simulink model "two_legged_raibert_hopper"  (R2014a)
settings: Solver=FixedStepDiscrete  StartTime=0.0  StopTime=inf  FixedStep=sample_time  RelTol=1e-3
undefined symbols (not defined in the file): A1_notch_f1, A2_notch_f1, A_lpf_accel, A_lpf_dtau, B1_lpf_accel, B1_lpf_dtau, B1_notch_f1, B2_lpf_accel, B2_lpf_dtau, B2_notch_f1, boom_height, boom_mount_angle, boom_mount_to_center_diagonal, boom_mount_to_com, contact_threshold, control_start_time, desired_torso_angle, DiscIntNeverNeededParam, dt_thrust, dx_avg_desired, dx_avg_samples, dx_desired_step, extra_leg_damping, F_thrust, fcut_contact, g, i_limit_lateral, initial_dt, j_segments, k_ff, K_notch_f1, k_placement, k_sea, kd_flight, kd_lateral, kd_leg_angle, kd_leg_length_secondary, kd_sea_torque_flight, kd_sea_torque_stance, kd_torso, kd_virtual, ki_lateral, kp_flight_max, kp_flight_min, kp_lateral, kp_leg_angle, kp_leg_length_secondary, kp_sea_torque_flight, kp_sea_torque_stance, kp_torso, kp_virtual, l0_virtual, l_boom, l_max, l_min, l_retract, l_seg, lambda1, lambda2, lateral_offset ... (+20)
libraries: simulink x14
(part 1 of 2)
settings Model: xpc_rtwmakecfg_data=_xpcethercatlib_  BufferReuse=off  Creator=wmartin  LastModifiedBy=wmartin
settings SolverCC: EnableConcurrentExecution=on
settings DataIOCC: MaxDataPoints=1000000000  SaveFormat=StructureWithTime
settings OptimizationCC: BlockReduction=off  OptimizeBlockIOStorage=off  BufferReuse=off  GlobalBufferReuse=off  ExpressionFolding=off  ExpressionDepthLimit=2147483647  LocalBlockOutputs=off
settings DebuggingCC: UnderspecifiedInitializationDetection=Classic  StateNameClashWarn=warning
settings HardwareCC: ProdIntDivRoundTo=Zero  ProdEndianess=LittleEndian  ProdHWDeviceType=Generic->32-bit x86 compatible
settings RTWCC: SystemTargetFile=slrt.tlc  TemplateMakefile=slrt_default_tmf  Description=Simulink Real-Time  RTWVerbose=off  ProcessScript=slrt_make_rtw_hook  RTWCompilerOptimization=On
settings SimulinkRealTimeCC: GeneratePreprocessorConditionals=Disable all  EnableShiftOperators=on  RL32LogBufSizeModifier=100000000

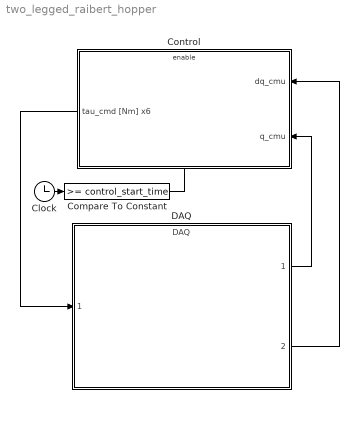
== system two_legged_raibert_hopper ==
  Clock : Clock
  Compare To Constant : simulink/Logic and Bit Operations/Compare To Constant  relop=>=  const=control_start_time  OutDataTypeStr=boolean
  Control : Subsystem
  DAQ : ModelReference  ModelNameDialog=DAQ  SimulationMode=Normal  ModelReferenceVersion=1.1402  CopyOfModelName=DAQ  DefaultDataLogging=on
  wires:
  DAQ/1 -> Control/2(q_cmu)
  DAQ/2 -> Control/1(dq_cmu)
  Clock/1 -> Compare To Constant/1
  Compare To Constant/1 -> Control/Enable
  Control/1(tau_cmd [Nm] x6) -> DAQ/1

== system two_legged_raibert_hopper/Control ==
  dq_cmu : Inport
  q_cmu : Inport  Port=2
  Enable : EnablePort  StatesWhenEnabling=reset
  Actuator Control : Subsystem
  Behavior Control : Subsystem
  tau_cmd [Nm] x6 : Outport  InitialOutput=[0 0 0 0 0 0]
  wires:
  Behavior Control/1(motor_torque_cmd) -> Actuator Control/1(tau_desired [Nm] x6)
  dq_cmu/1 -> Actuator Control/3(dq_cmu), Behavior Control/1(dq_cmu)
  Actuator Control/1(tau_cmd [Nm] x6) -> tau_cmd [Nm] x6/1
  q_cmu/1 -> Behavior Control/2(q_cmu), Actuator Control/2(q_cmu)

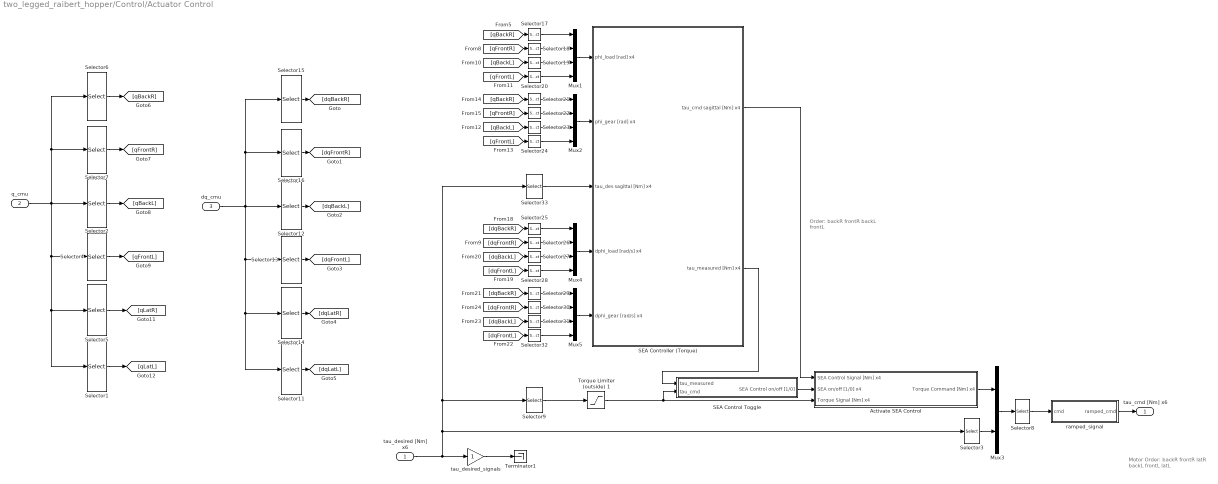
== system two_legged_raibert_hopper/Control/Actuator Control ==
  note: Motor Order:
      |
      | backR
      | frontR
      | latR
      | backL
      | frontL
      | latL
  note: Order:
      | backR
      | frontR
      | backL
      | frontL
  tau_desired [Nm] x6 : Inport
  q_cmu : Inport  Port=2
  dq_cmu : Inport  Port=3
  Activate SEA Control : Subsystem
  Mux{1..2,4..5} (4 alike) : Mux
  Mux3 : Mux  Inputs=2
  SEA Control Toggle : Subsystem
  SEA Controller (Torque) : Subsystem
  Selector1 : Selector  InputPortWidth=13  Indices=[10]
  Selector11 : Selector  InputPortWidth=13  Indices=[10]
  Selector12 : Selector  InputPortWidth=13  Indices=[5 6]
  Selector13 : Selector  InputPortWidth=13  Indices=[7 8]
  Selector14 : Selector  InputPortWidth=13  Indices=[9]
  Selector15 : Selector  InputPortWidth=13  Indices=[1 2]
  Selector16 : Selector  InputPortWidth=13  Indices=[3 4]
  Selector{17..20,25..28} (8 alike) : Selector  InputPortWidth=2  Indices=[1]
  Selector2 : Selector  InputPortWidth=13  Indices=[5 6]
  Selector{21..24,29..32} (8 alike) : Selector  InputPortWidth=2  Indices=[2]
  Selector3 : Selector  InputPortWidth=6  Indices=[3 6]
  Selector33 : Selector  InputPortWidth=6  Indices=[1 2 4 5]
  Selector4 : Selector  InputPortWidth=13  Indices=[7 8]
  Selector5 : Selector  InputPortWidth=13  Indices=[9]
  Selector6 : Selector  InputPortWidth=13  Indices=[1 2]
  Selector7 : Selector  InputPortWidth=13  Indices=[3 4]
  Selector8 : Selector  InputPortWidth=6  Indices=[1 2 5 3 4 6]
  Selector9 : Selector  InputPortWidth=6  Indices=[1 2 4 5]
  Terminator1 : Terminator
  Torque Limiter (outside) 1 : Saturate  UpperLimit=max_sagittal_unloaded_torque  LowerLimit=-max_sagittal_unloaded_torque
      settings: AttributesFormatString=Hi: %<UpperLimit>\nLo: %<LowerLimit>
  ramped_signal : Subsystem
  tau_desired_signals : Gain  Description=xPCTag(1)=tau_cmd_signal;
  tau_cmd [Nm] x6 : Outport  InitialOutput=[0 0 0 0 0 0]
  wires:
  Mux3/1 -> Selector8/1
  Selector3/1 -> Mux3/2
  Selector33/1 -> SEA Controller (Torque)/3(tau_des sagittal [Nm] x4)
  [dqFrontL] -> Selector32/1
  [dqBackL] -> Selector31/1
  [dqFrontR] -> Selector30/1
  Selector32/1 -> Mux5/4
  Selector30/1 -> Mux5/2
  Selector31/1 -> Mux5/3
  Selector29/1 -> Mux5/1
  [dqBackR] -> Selector29/1
  Mux5/1 -> SEA Controller (Torque)/5(dphi_gear [rad/s] x4)
  [dqFrontL] -> Selector28/1
  [dqBackL] -> Selector27/1
  [dqFrontR] -> Selector26/1
  Selector28/1 -> Mux4/4
  Selector26/1 -> Mux4/2
  Selector27/1 -> Mux4/3
  Selector25/1 -> Mux4/1
  [dqBackR] -> Selector25/1
  Mux4/1 -> SEA Controller (Torque)/4(dphi_load [rad/s] x4)
  [qFrontL] -> Selector24/1
  [qBackL] -> Selector23/1
  [qFrontR] -> Selector22/1
  Selector24/1 -> Mux2/4
  Selector22/1 -> Mux2/2
  Selector23/1 -> Mux2/3
  Selector21/1 -> Mux2/1
  [qBackR] -> Selector21/1
  Mux2/1 -> SEA Controller (Torque)/2(phi_gear [rad] x4)
  [qFrontL] -> Selector20/1
  [qBackL] -> Selector19/1
  [qFrontR] -> Selector18/1
  Selector20/1 -> Mux1/4
  Selector18/1 -> Mux1/2
  Selector19/1 -> Mux1/3
  Selector17/1 -> Mux1/1
  [qBackR] -> Selector17/1
  Mux1/1 -> SEA Controller (Torque)/1(phi_load [rad] x4)
  Selector13/1 -> [dqFrontL]
  Selector12/1 -> [dqBackL]
  Selector16/1 -> [dqFrontR]
  Selector15/1 -> [dqBackR]
  Selector11/1 -> [dqLatL]
  Selector14/1 -> [dqLatR]
  dq_cmu/1 -> Selector11/1, Selector14/1, Selector13/1, Selector15/1, Selector16/1, Selector12/1
  Selector8/1 -> ramped_signal/1(cmd)
  q_cmu/1 -> Selector2/1, Selector7/1, Selector6/1, Selector4/1, Selector5/1, Selector1/1
  Selector4/1 -> [qFrontL]
  Selector2/1 -> [qBackL]
  Selector7/1 -> [qFrontR]
  Selector6/1 -> [qBackR]
  Selector1/1 -> [qLatL]
  Selector5/1 -> [qLatR]
  tau_desired_signals/1 -> Terminator1/1
  ramped_signal/1(ramped_cmd) -> tau_cmd [Nm] x6/1
  tau_desired [Nm] x6/1 -> Selector33/1, Selector9/1, Selector3/1, tau_desired_signals/1
  Activate SEA Control/1(Torque Command [Nm] x4) -> Mux3/1
  Torque Limiter (outside) 1/1 -> Activate SEA Control/3(Torque Signal [Nm] x4), SEA Control Toggle/2(tau_cmd)
  SEA Controller (Torque)/1(tau_cmd sagittal [Nm] x4) -> Activate SEA Control/1(SEA Control Signal [Nm] x4)
  SEA Control Toggle/1(SEA Control on/off [1/0]) -> Activate SEA Control/2("SEA on/off [1/0] x4 ")
  SEA Controller (Torque)/2(tau_measured [Nm] x4) -> SEA Control Toggle/1(tau_measured)
  Selector9/1 -> Torque Limiter (outside) 1/1

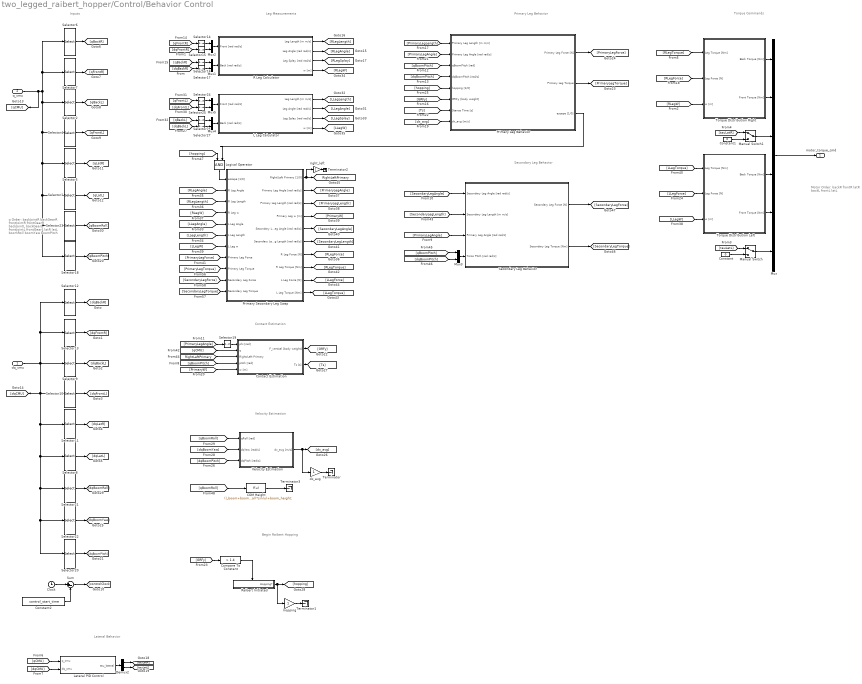
== system two_legged_raibert_hopper/Control/Behavior Control ==
  note: Motor Order:
      |
      | backR
      | frontR
      | latR
      | backL
      | frontL
      | latL
  note: q Order:
      |
      | backJointR
      | backGearR
      | frontJointR
      | frontGearR
      |
      | backJointL
      | backGearL
      | frontJointL
      | frontGearL
      |
      | latR
      | latL
      |
      | boomRoll
      | boomYaw
      | boomPitch
  note: Inputs
  note: Primary Leg Behavior
  note: Secondary Leg Behavior
  note: Torque Commands
  note: Lateral Behavior
  note: Leg Measurements
  note: Contact Estimation
  note: Velocity Estimation
  note: Begin Raibert Hopping
  dq_cmu : Inport
  q_cmu : Inport  Port=2
  COM Height : Fcn  Expr=(l_boom+boom_mount_to_center_diagonal)*sin(u)+boom_height;
  Clock : Clock
  Compare To Constant : simulink/Logic and Bit Operations/Compare To Constant  relop=>  const=1.4  OutDataTypeStr=boolean
  Constant : Constant  Value=0
  Constant1 : Constant  Value=0
  Constant2 : Constant  Value=control_start_time
  Contact Estimation : Subsystem
  Demux2 : Demux  Outputs=2
  L Leg Calculator : Subsystem
  Lateral PID Control : Subsystem
  Logical Operator : Logic  IconShape=distinctive  AllPortsSameDT=off  OutDataTypeStr=boolean
  Manual Switch : ManualSwitch
  Manual Switch1 : ManualSwitch
  Mux : Mux  Inputs=6
  Mux{1..5} (5 alike) : Mux  Inputs=2
  Primary Leg Behavior : Subsystem
  Primary Secondary Leg Swap : Subsystem
  R Leg Calculator : Subsystem
  Raibert Initiated : Subsystem
  Secondary Leg Behavior : Subsystem
  Selector1 : Selector  InputPortWidth=13  Indices=[10]
  Selector10 : Selector  InputPortWidth=13  Indices=[7 8]
  Selector11 : Selector  InputPortWidth=13  Indices=[9]
  Selector12 : Selector  InputPortWidth=13  Indices=[1 2]
  Selector13 : Selector  InputPortWidth=13  Indices=[3 4]
  Selector{14..17,19,24..27} (9 alike) : Selector  InputPortWidth=2  Indices=[1]
  Selector18 : Selector  InputPortWidth=13  Indices=[13]
  Selector2 : Selector  InputPortWidth=13  Indices=[5 6]
  Selector20 : Selector  InputPortWidth=13  Indices=[13]
  Selector21 : Selector  InputPortWidth=13  Indices=[11]
  Selector22 : Selector  InputPortWidth=13  Indices=[12]
  Selector23 : Selector  InputPortWidth=13  Indices=[11]
  Selector4 : Selector  InputPortWidth=13  Indices=[7 8]
  Selector5 : Selector  InputPortWidth=13  Indices=[9]
  Selector6 : Selector  InputPortWidth=13  Indices=[1 2]
  Selector7 : Selector  InputPortWidth=13  Indices=[3 4]
  Selector8 : Selector  InputPortWidth=13  Indices=[10]
  Selector9 : Selector  InputPortWidth=13  Indices=[5 6]
  Sum : Sum  Inputs=|+-
  Terminator{,1..3} (4 alike) : Terminator
  Torque Distribution Left : Subsystem
  Torque Distribution Right : Subsystem
  Velocity Estimation : Subsystem
  dx_avg : Gain
  hopping : Gain
  right_left : Gain
  motor_torque_cmd : Outport  OutputWhenDisabled=reset  InitialOutput=[0 0 0 0 0 0]
  tag scope: RightLeftPrimary=global
  wires:
  Lateral PID Control/1(tau_lateral) -> Demux2/1
  [dqCMU] -> Lateral PID Control/2(dq_cmu)
  [qCMU] -> Lateral PID Control/1(q_cmu)
  Sum/1 -> [controlClock]
  Selector4/1 -> [qFrontL]
  Selector2/1 -> [qBackL]
  Selector7/1 -> [qFrontR]
  Selector6/1 -> [qBackR]
  Selector1/1 -> [qLatL]
  Selector5/1 -> [qLatR]
  Constant2/1 -> Sum/2
  Clock/1 -> Sum/1
  Constant1/1 -> Manual Switch1/2
  Constant/1 -> Manual Switch/2
  Manual Switch/1 -> Mux/6
  Manual Switch1/1 -> Mux/3
  Mux/1 -> motor_torque_cmd/1
  Selector8/1 -> [dqLatL]
  Selector11/1 -> [dqLatR]
  Selector12/1 -> [dqBackR]
  Selector13/1 -> [dqFrontR]
  Selector9/1 -> [dqBackL]
  Selector10/1 -> [dqFrontL]
  [qBackR] -> Selector16/1
  [dqBackR] -> Selector17/1
  [qFrontR] -> Selector14/1
  [dqFrontR] -> Selector15/1
  Mux2/1 -> R Leg Calculator/1(Front [rad rad/s])
  Mux1/1 -> R Leg Calculator/2(Back [rad rad/s])
  R Leg Calculator/1("Leg Length [m m/s] ") -> [RLegLength]
  R Leg Calculator/2(Leg Angle [rad rad/s]) -> [RLegAngle]
  R Leg Calculator/3(Leg Splay [rad rad/s]) -> [RLegSplay]
  Torque Distribution Right/1(Back Torque [Nm]) -> Mux/1
  Torque Distribution Right/2(Front Torque [Nm]) -> Mux/2
  Demux2/1 -> [tauLatR]
  Demux2/2 -> [tauLatL]
  [tauLatR] -> Manual Switch1/1
  [tauLatL] -> Manual Switch/1
  [RLegW] -> Torque Distribution Right/3(w [m])
  Selector14/1 -> Mux2/1
  Selector15/1 -> Mux2/2
  Selector17/1 -> Mux1/2
  Selector16/1 -> Mux1/1
  [PrimaryW] -> Contact Estimation/5(w [m])
  q_cmu/1 -> Selector6/1, Selector7/1, Selector2/1, Selector4/1, Selector5/1, Selector18/1, Selector23/1, Selector1/1, [qCMU]
  Selector18/1 -> [qBoomPitch]
  [qBoomPitch] -> Contact Estimation/4(pitch [rad])
  [PrimaryLegAngle] -> Selector19/1
  Selector19/1 -> Contact Estimation/1(phi [rad])
  Contact Estimation/1(F_vertical [body weight]) -> [GRFy]
  Selector20/1 -> [dqBoomPitch]
  [RLegForce] -> Torque Distribution Right/2(Leg Force [N])
  [RLegTorque] -> Torque Distribution Right/1(Leg Torque [Nm])
  Selector22/1 -> [dqBoomYaw]
  Contact Estimation/2(Ts [s]) -> [Ts]
  [GRFy] -> Compare To Constant/1
  Raibert Initiated/1(Hopping?) -> hopping/1, [hopping]
  dq_cmu/1 -> Selector20/1, Selector22/1, Selector21/1, Selector8/1, Selector11/1, Selector10/1, [dqCMU], Selector12/1, Selector13/1, Selector9/1
  Selector21/1 -> [dqBoomRoll]
  Selector23/1 -> [qBoomRoll]
  [qBackL] -> Selector26/1
  [dqBackL] -> Selector27/1
  [qFrontL] -> Selector24/1
  [dqFrontL] -> Selector25/1
  Mux5/1 -> L Leg Calculator/1(Front [rad rad/s])
  Mux4/1 -> L Leg Calculator/2(Back [rad rad/s])
  L Leg Calculator/1("Leg Length [m m/s] ") -> [LLegLength]
  L Leg Calculator/2(Leg Angle [rad rad/s]) -> [LLegAngle]
  L Leg Calculator/3(Leg Splay [rad rad/s]) -> [LLegSplay]
  Selector24/1 -> Mux5/1
  Selector25/1 -> Mux5/2
  Selector27/1 -> Mux4/2
  Selector26/1 -> Mux4/1
  R Leg Calculator/4(w [m]) -> [RLegW]
  L Leg Calculator/4(w [m]) -> [LLegW]
  [LLegAngle] -> Primary Secondary Leg Swap/5(L Leg Angle)
  [LLegLength] -> Primary Secondary Leg Swap/6(L Leg Length)
  [LLegW] -> Primary Secondary Leg Swap/7(L Leg w)
  [RLegAngle] -> Primary Secondary Leg Swap/2(R Leg Angle)
  [RLegLength] -> Primary Secondary Leg Swap/3(R Leg Length)
  [RLegW] -> Primary Secondary Leg Swap/4(R Leg w)
  [PrimaryLegForce] -> Primary Secondary Leg Swap/8(Primary Leg Force)
  [PrimaryLegTorque] -> Primary Secondary Leg Swap/9(Primary Leg Torque)
  [SecondaryLegForce] -> Primary Secondary Leg Swap/10(Secondary Leg Force)
  [SecondaryLegTorque] -> Primary Secondary Leg Swap/11(Secondary Leg Torque)
  Primary Secondary Leg Swap/5(Secondary Leg Angle [rad rad/s]) -> [SecondaryLegAngle]
  Primary Secondary Leg Swap/6(Secondary Leg Length [rad rad/s]) -> [SecondaryLegLength]
  Primary Secondary Leg Swap/2(Primary Leg Angle [rad rad/s]) -> [PrimaryLegAngle]
  Primary Secondary Leg Swap/3(Primary Leg Length [rad rad/s]) -> [PrimaryLegLength]
  Primary Secondary Leg Swap/4(Primary Leg w [m]) -> [PrimaryW]
  Primary Secondary Leg Swap/7(R Leg Force [N]) -> [RLegForce]
  Primary Secondary Leg Swap/8(R Leg Torque [Nm]) -> [RLegTorque]
  Primary Secondary Leg Swap/9(L Leg Force [N]) -> [LLegForce]
  Primary Secondary Leg Swap/10(L Leg Torque [Nm]) -> [LLegTorque]
  Primary Leg Behavior/3(escape [1/0]) -> Logical Operator/2
  Primary Secondary Leg Swap/1(Right/Left Primary [1/0]) -> right_left/1, [RightLeftPrimary]
  [PrimaryLegLength] -> Primary Leg Behavior/1(Primary Leg Length [m m/s])
  [hopping] -> Primary Leg Behavior/5(hopping [1/0])
  [GRFy] -> Primary Leg Behavior/6(GRFy [body weight])
  [qBoomPitch] -> Primary Leg Behavior/3(qBoomPitch [rad])
  [dqBoomPitch] -> Primary Leg Behavior/4(dqBoomPitch [rad/s])
  [PrimaryLegAngle] -> Primary Leg Behavior/2(Primary Leg Angle [rad rad/s])
  [Ts] -> Primary Leg Behavior/7(Stance Time [s])
  [dx_avg] -> Primary Leg Behavior/8(dx_avg [m/s])
  Primary Leg Behavior/1(Primary Leg Force [N]) -> [PrimaryLegForce]
  Primary Leg Behavior/2(Primary Leg Torque) -> [PrimaryLegTorque]
  Velocity Estimation/1(dx_avg [m/s]) -> dx_avg/1, [dx_avg]
  [qBoomRoll] -> Velocity Estimation/1(qRoll [rad])
  [dqBoomYaw] -> Velocity Estimation/2(dqYaw [rad/s])
  [dqBoomPitch] -> Velocity Estimation/3(dqPitch [rad/s])
  dx_avg/1 -> Terminator/1
  hopping/1 -> Terminator1/1
  Torque Distribution Left/1(Back Torque [Nm]) -> Mux/4
  Torque Distribution Left/2(Front Torque [Nm]) -> Mux/5
  [LLegTorque] -> Torque Distribution Left/1(Leg Torque [Nm])
  [LLegForce] -> Torque Distribution Left/2(Leg Force [N])
  [LLegW] -> Torque Distribution Left/3(w [m])
  [qCMU] -> Contact Estimation/2(q)
  [RightLeftPrimary] -> Contact Estimation/3(Right/Left Primary)
  Secondary Leg Behavior/1(Secondary Leg Force [N]) -> [SecondaryLegForce]
  Secondary Leg Behavior/2(Secondary Leg Torque [Nm]) -> [SecondaryLegTorque]
  [PrimaryLegAngle] -> Secondary Leg Behavior/3(Primary Leg Angle [rad rad/s])
  [SecondaryLegAngle] -> Secondary Leg Behavior/1(Secondary Leg Angle [rad rad/s])
  [SecondaryLegLength] -> Secondary Leg Behavior/2(Secondary Leg Length [m m/s])
  [qBoomPitch] -> Mux3/1
  [dqBoomPitch] -> Mux3/2
  Mux3/1 -> Secondary Leg Behavior/4(Torso Pitch [rad rad/s])
  right_left/1 -> Terminator2/1
  [hopping] -> Logical Operator/1
  Logical Operator/1 -> Primary Secondary Leg Swap/1(escape [1/0])
  [qBoomRoll] -> COM Height/1
  COM Height/1 -> Terminator3/1
  Compare To Constant/1 -> Raibert Initiated/Enable

== system two_legged_raibert_hopper/Control/Actuator Control/Activate SEA Control ==
  SEA Control Signal [Nm] x4 : Inport
  "SEA on/off [1/0] x4 " : Inport  Port=2
  Torque Signal [Nm] x4 : Inport  Port=3
  Demux : Demux
  Demux2 : Demux
  Demux3 : Demux
  Mux6 : Mux
  Switch{,1..3} (4 alike) : Switch  Criteria=u2 ~= 0
  Torque Command [Nm] x4 : Outport
  wires:
  Demux2/2 -> Switch1/3
  Demux2/1 -> Switch/3
  Demux/1 -> Switch/1
  Switch/1 -> Mux6/1
  Switch1/1 -> Mux6/2
  Switch3/1 -> Mux6/4
  Demux3/1 -> Switch/2
  Mux6/1 -> Torque Command [Nm] x4/1
  Demux3/3 -> Switch2/2
  Demux3/2 -> Switch1/2
  Demux/3 -> Switch2/1
  Switch2/1 -> Mux6/3
  Demux/4 -> Switch3/1
  Demux2/4 -> Switch3/3
  Demux3/4 -> Switch3/2
  Demux/2 -> Switch1/1
  Demux2/3 -> Switch2/3
  SEA Control Signal [Nm] x4/1 -> Demux/1
  "SEA on/off [1/0] x4 "/1 -> Demux3/1
  Torque Signal [Nm] x4/1 -> Demux2/1

== system two_legged_raibert_hopper/Control/Actuator Control/SEA Control Toggle ==
  tau_measured : Inport
  tau_cmd : Inport  Port=2
  Abs : Abs
  Abs1 : Abs
  But Commanding a Small Torque? : simulink/Logic and Bit Operations/Compare To Constant  relop=<  const=sea_control_torque_cmd_small_threshold  OutDataTypeStr=boolean
  Logical Operator1 : Logic  AllPortsSameDT=off  OutDataTypeStr=boolean
  Logical Operator2 : Logic  Operator=NOT  AllPortsSameDT=off  OutDataTypeStr=boolean
  Measuring a Large Torque? (High Gains) : simulink/Logic and Bit Operations/Compare To Constant  relop=>=  const=stance_flight_torque_threshold  OutDataTypeStr=boolean
  SEA Control on/off [1/0] : Outport
  wires:
  Logical Operator2/1 -> SEA Control on/off [1/0]/1
  But Commanding a Small Torque?/1 -> Logical Operator1/2
  Logical Operator1/1 -> Logical Operator2/1
  tau_cmd/1 -> Abs/1
  Abs/1 -> But Commanding a Small Torque?/1
  tau_measured/1 -> Abs1/1
  Measuring a Large Torque? (High Gains)/1 -> Logical Operator1/1
  Abs1/1 -> Measuring a Large Torque? (High Gains)/1

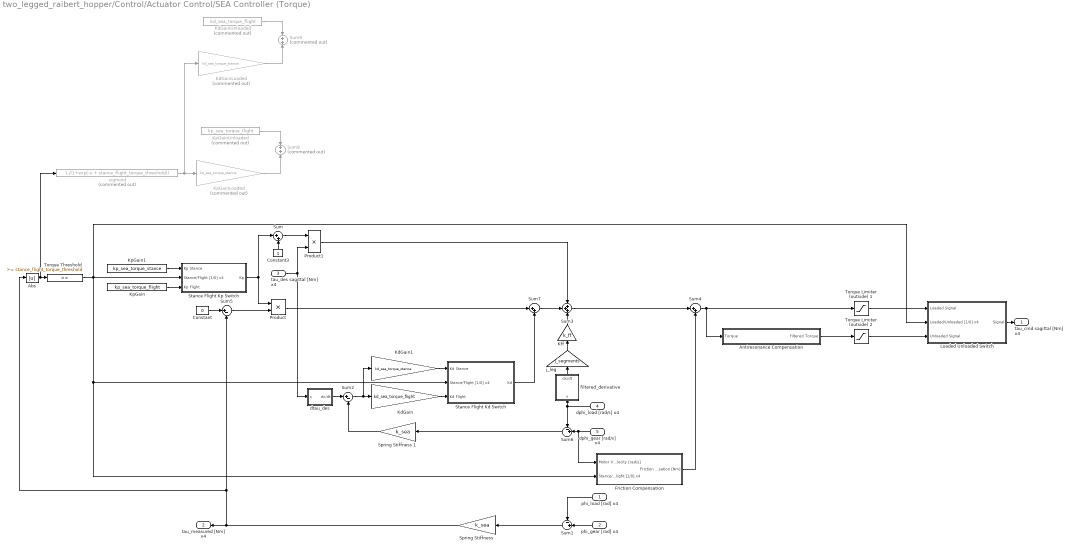
== system two_legged_raibert_hopper/Control/Actuator Control/SEA Controller (Torque) ==
  phi_load [rad] x4 : Inport
  phi_gear [rad] x4 : Inport  Port=2
  tau_des sagittal [Nm] x4 : Inport  Port=3
  dphi_load [rad/s] x4 : Inport  Port=4
  dphi_gear [rad/s] x4 : Inport  Port=5
  Abs : Abs
  Antiresonance Compensation : Subsystem
  Constant : Constant  Value=0
  Constant3 : Constant
  Friction Compensation : Subsystem
  KdGain : Gain  Description=xPCTag(1)=kd_sea_torque;  Gain=kd_sea_torque_flight
  KdGain1 : Gain  Description=xPCTag(1)=kd_sea_torque;  Gain=kd_sea_torque_stance
  KdGainLoaded : Gain  Description=xPCTag(1)=kd_sea_torque;  Commented=on  Gain=kd_sea_torque_stance
  KdGainUnloaded : Constant  Commented=on  Value=kd_sea_torque_flight  SampleTime=sample_time
  Kff : Gain  Gain=k_ff
  KpGain : Constant  Value=kp_sea_torque_flight  SampleTime=sample_time
  KpGain1 : Constant  Value=kp_sea_torque_stance  SampleTime=sample_time
  KpGainLoaded : Gain  Description=xPCTag(1)=kd_sea_torque;  Commented=on  Gain=kp_sea_torque_stance
  KpGainUnloaded : Constant  Commented=on  Value=kp_sea_torque_flight  SampleTime=sample_time
  Loaded Unloaded Switch : Subsystem
  Product : Product  SampleTime=sample_time  RndMeth=Zero
  Product1 : Product  RndMeth=Zero
  Spring Stiffness : Gain  Gain=k_sea
  Spring Stiffness 1 : Gain  Gain=k_sea
  Stance Flight Kd Switch : Subsystem
  Stance Flight Kp Switch : Subsystem
  Sum : Sum  Inputs=|++  SampleTime=sample_time
  Sum1 : Sum  Inputs=-+|
  Sum2 : Sum  Inputs=|+-
  Sum3 : Sum  Inputs=+++
  Sum4 : Sum  Inputs=|++
  Sum5 : Sum  Inputs=|+-
  Sum6 : Sum  Inputs=-+|
  Sum7 : Sum  Inputs=|++
  Sum8 : Sum  Commented=on  Inputs=+|+  SampleTime=sample_time
  Sum9 : Sum  Commented=on  Inputs=+|+  SampleTime=sample_time
  Torque Limiter (outside) 1 : Saturate  UpperLimit=max_sagittal_loaded_torque  LowerLimit=-max_sagittal_loaded_torque
      settings: AttributesFormatString=Hi: %<UpperLimit>\nLo: %<LowerLimit>
  Torque Limiter (outside) 2 : Saturate  UpperLimit=max_sagittal_unloaded_torque  LowerLimit=-max_sagittal_unloaded_torque
      settings: AttributesFormatString=Hi: %<UpperLimit>\nLo: %<LowerLimit>
  Torque Threshold : simulink/Logic and Bit Operations/Compare To Constant  relop=>=  const=stance_flight_torque_threshold  OutDataTypeStr=boolean
  dtau_des : Subsystem
  filtered_derivative : Subsystem
  j_leg : Gain  Description=xPCTag(1)=kd_sea_torque;  Gain=j_segments
  sigmoid : Fcn  Commented=on  Expr=1./(1+exp(-u + stance_flight_torque_threshold))
  tau_cmd sagittal [Nm] x4 : Outport
  tau_measured [Nm] x4 : Outport  Port=2
  wires:
  Antiresonance Compensation/1(Filtered Torque) -> Torque Limiter (outside) 2/1
  Sum3/1 -> Sum4/1
  Sum7/1 -> Sum3/2
  Product1/1 -> Sum3/1
  Sum4/1 -> Antiresonance Compensation/1(Torque), Torque Limiter (outside) 1/1
  Stance Flight Kd Switch/1(Kd) -> Sum7/2
  Abs/1 -> sigmoid/1, Torque Threshold/1
  Stance Flight Kp Switch/1(Kp) -> Product/1, Sum/1
  Spring Stiffness/1 -> tau_measured [Nm] x4/1, Abs/1, Sum5/2
  KdGain1/1 -> Stance Flight Kd Switch/1(Kd Stance)
  KpGain/1 -> Stance Flight Kp Switch/3(Kp Flight)
  Torque Threshold/1 -> Loaded Unloaded Switch/2(Loaded/Unloaded [1/0] x4), Stance Flight Kp Switch/2(Stance/Flight [1/0] x4), Friction Compensation/2(Stance/Flight [1/0] x4), Stance Flight Kd Switch/2(Stance/Flight [1/0] x4)
  KpGain1/1 -> Stance Flight Kp Switch/1(Kp Stance)
  Sum1/1 -> Spring Stiffness/1
  phi_load [rad] x4/1 -> Sum1/1
  phi_gear [rad] x4/1 -> Sum1/2
  Constant/1 -> Sum5/1
  dtau_des/1(dx/dt) -> Sum2/1
  Sum6/1 -> Spring Stiffness 1/1
  Spring Stiffness 1/1 -> Sum2/2
  dphi_load [rad/s] x4/1 -> Sum6/1, filtered_derivative/1(x)
  dphi_gear [rad/s] x4/1 -> Friction Compensation/1(Motor Velocity [rad/s]), Sum6/2
  Sum2/1 -> KdGain/1, KdGain1/1
  Sum5/1 -> Product/2
  Product/1 -> Sum7/1
  KdGain/1 -> Stance Flight Kd Switch/3(Kd Flight)
  Constant3/1 -> Sum/2
  Sum/1 -> Product1/1
  filtered_derivative/1(dx/dt) -> j_leg/1
  j_leg/1 -> Kff/1
  Torque Limiter (outside) 1/1 -> Loaded Unloaded Switch/1(Loaded Signal)
  Kff/1 -> Sum3/3
  tau_des sagittal [Nm] x4/1 -> dtau_des/1(x), Product1/2
  Friction Compensation/1(Friction Compensation [Nm]) -> Sum4/2
  Torque Limiter (outside) 2/1 -> Loaded Unloaded Switch/3(Unloaded Signal)
  Loaded Unloaded Switch/1(Signal) -> tau_cmd sagittal [Nm] x4/1
  sigmoid/1 -> KdGainLoaded/1, KpGainLoaded/1
  KpGainUnloaded/1 -> Sum8/1
  KpGainLoaded/1 -> Sum8/2
  KdGainUnloaded/1 -> Sum9/1
  KdGainLoaded/1 -> Sum9/2

== system two_legged_raibert_hopper/Control/Actuator Control/ramped_signal ==
  cmd : Inport
  Demux : Demux
  Mux1 : Mux
  Mux6 : Mux  Inputs=2
  Product : Product  RndMeth=Zero
  Product1 : Product  RndMeth=Zero
  Ramp : simulink/Sources/Ramp  slope=1/sagittal_torque_ramp_time  start=sagittal_starting_time  X0=0
      settings: AttributesFormatString=Start: %<start>\nSlope: %<slope>
  Ramp1 : simulink/Sources/Ramp  slope=1/lateral_torque_ramp_time  start=control_start_time  X0=0
      settings: AttributesFormatString=Start: %<start>\nSlope: %<slope>
  Saturation : Saturate  UpperLimit=1  LowerLimit=0
      settings: AttributesFormatString=Hi: %<UpperLimit>\nLo: %<LowerLimit>
  Saturation1 : Saturate  UpperLimit=1  LowerLimit=0
      settings: AttributesFormatString=Hi: %<UpperLimit>\nLo: %<LowerLimit>
  Selector10 : Selector  InputPortWidth=6  Indices=[1 2 4 5]
  Selector34 : Selector  InputPortWidth=6  Indices=[1 2 5 3 4 6]
  Selector9 : Selector  InputPortWidth=6  Indices=[3 6]
  ramped_cmd : Outport
  wires:
  Selector9/1 -> Product1/1
  Saturation1/1 -> Product1/2
  Ramp1/1 -> Saturation1/1
  Saturation/1 -> Product/2
  Ramp/1 -> Saturation/1
  Product/1 -> Mux6/1
  cmd/1 -> Selector10/1, Selector9/1
  Product1/1 -> Mux6/2
  Selector34/1 -> ramped_cmd/1
  Selector10/1 -> Demux/1
  Mux6/1 -> Selector34/1
  Demux/1 -> Mux1/1
  Demux/2 -> Mux1/2
  Mux1/1 -> Product/1
  Demux/4 -> Mux1/4
  Demux/3 -> Mux1/3

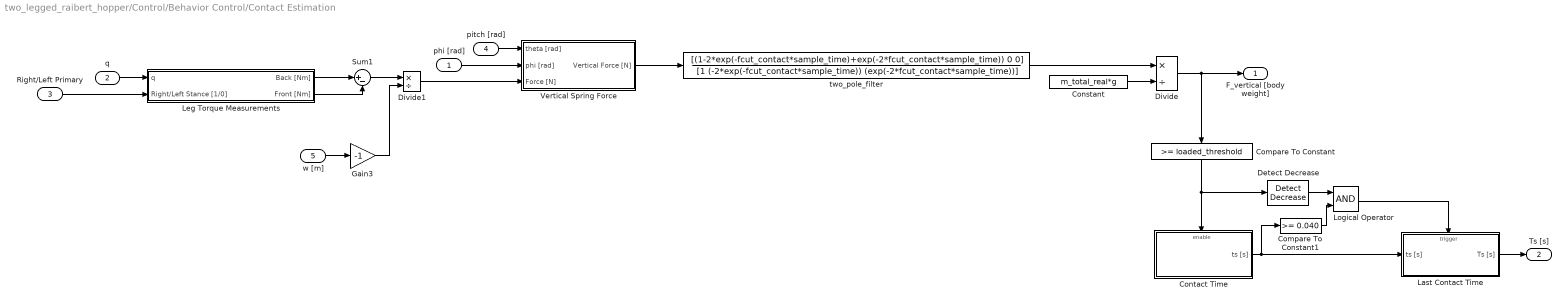
== system two_legged_raibert_hopper/Control/Behavior Control/Contact Estimation ==
  phi [rad] : Inport
  q : Inport  Port=2
  Right/Left Primary : Inport  Port=3
  pitch [rad] : Inport  Port=4
  w [m] : Inport  Port=5
  Compare To Constant : simulink/Logic and Bit Operations/Compare To Constant  relop=>=  const=loaded_threshold  OutDataTypeStr=boolean
  Compare To Constant1 : simulink/Logic and Bit Operations/Compare To Constant  relop=>=  const=0.040  OutDataTypeStr=boolean
  Constant : Constant  Value=m_total_real*g
  Contact Time : Subsystem
  Detect Decrease : simulink/Logic and Bit Operations/Detect Decrease  vinit=0.0  InputProcessing=Inherited  OutDataTypeStr=boolean
  Divide : Product  Inputs=*/
  Divide1 : Product  Inputs=*/
  Gain3 : Gain  Gain=-1
  Last Contact Time : Subsystem
  Leg Torque Measurements : Subsystem
  Logical Operator : Logic  AllPortsSameDT=off  OutDataTypeStr=boolean
  Sum1 : Sum  Inputs=|+-
  Vertical Spring Force : Subsystem
  two_pole_filter : DiscreteTransferFcn  Numerator=[(1-2*exp(-fcut_contact*sample_time)+exp(-2*fcut_contact*sample_time)) 0 0]  Denominator=[1 (-2*exp(-fcut_contact*sample_time)) (exp(-2*fcut_contact*sample_time))]  SampleTime=sample_time
  F_vertical [body weight] : Outport
  Ts [s] : Outport  Port=2
  wires:
  Vertical Spring Force/1(Vertical Force [N]) -> two_pole_filter/1
  Constant/1 -> Divide/2
  two_pole_filter/1 -> Divide/1
  q/1 -> Leg Torque Measurements/1(q)
  Leg Torque Measurements/1(Back [Nm]) -> Sum1/1
  Leg Torque Measurements/2(Front [Nm]) -> Sum1/2
  Sum1/1 -> Divide1/1
  Divide1/1 -> Vertical Spring Force/3(Force [N])
  pitch [rad]/1 -> Vertical Spring Force/1(theta [rad])
  w [m]/1 -> Gain3/1
  Gain3/1 -> Divide1/2
  phi [rad]/1 -> Vertical Spring Force/2(phi [rad])
  Last Contact Time/1(Ts [s]) -> Ts [s]/1
  Contact Time/1(ts [s]) -> Last Contact Time/1(ts [s]), Compare To Constant1/1
  Compare To Constant/1 -> Detect Decrease/1, Contact Time/Enable
  Divide/1 -> F_vertical [body weight]/1, Compare To Constant/1
  Logical Operator/1 -> Last Contact Time/Trigger
  Detect Decrease/1 -> Logical Operator/1
  Compare To Constant1/1 -> Logical Operator/2
  Right/Left Primary/1 -> Leg Torque Measurements/2(Right/Left Stance [1/0])

== system two_legged_raibert_hopper/Control/Behavior Control/L Leg Calculator ==
  Front [rad rad/s] : Inport
  Back [rad rad/s] : Inport  Port=2
  Demux1 : Demux  Outputs=2
  Gain1 : Gain  Gain=2*l_seg
  Gain2 : Gain  Gain=l_seg
  Gain3 : Gain  Gain=-1
  Gain4 : Gain  Gain=0.5
  Gain5 : Gain  Gain=0.5
  Gain6 : Gain  Gain=2
  Mux1 : Mux  Inputs=2
  Product : Product  RndMeth=Zero
  Sum4 : Sum  Inputs=+|+
  Sum5 : Sum  Inputs=+|-
  Trigonometric Function : Trigonometry  Operator=cos
  Trigonometric Function1 : Trigonometry
  "Leg Length [m m/s] " : Outport
  Leg Angle [rad rad/s] : Outport  Port=2
  Leg Splay [rad rad/s] : Outport  Port=3
  w [m] : Outport  Port=4
  wires:
  Gain5/1 -> Leg Angle [rad rad/s]/1
  Sum4/1 -> Gain5/1
  Mux1/1 -> "Leg Length [m m/s] "/1
  Sum5/1 -> Demux1/1, Leg Splay [rad rad/s]/1
  Gain2/1 -> Gain6/1, Product/1
  Demux1/1 -> Gain4/1
  Gain3/1 -> Product/2
  Demux1/2 -> Gain3/1
  Back [rad rad/s]/1 -> Sum5/1, Sum4/1
  Front [rad rad/s]/1 -> Sum4/2, Sum5/2
  Product/1 -> Mux1/2
  Trigonometric Function1/1 -> Gain2/1
  Gain1/1 -> Mux1/1
  Trigonometric Function/1 -> Gain1/1
  Gain4/1 -> Trigonometric Function/1, Trigonometric Function1/1
  Gain6/1 -> w [m]/1

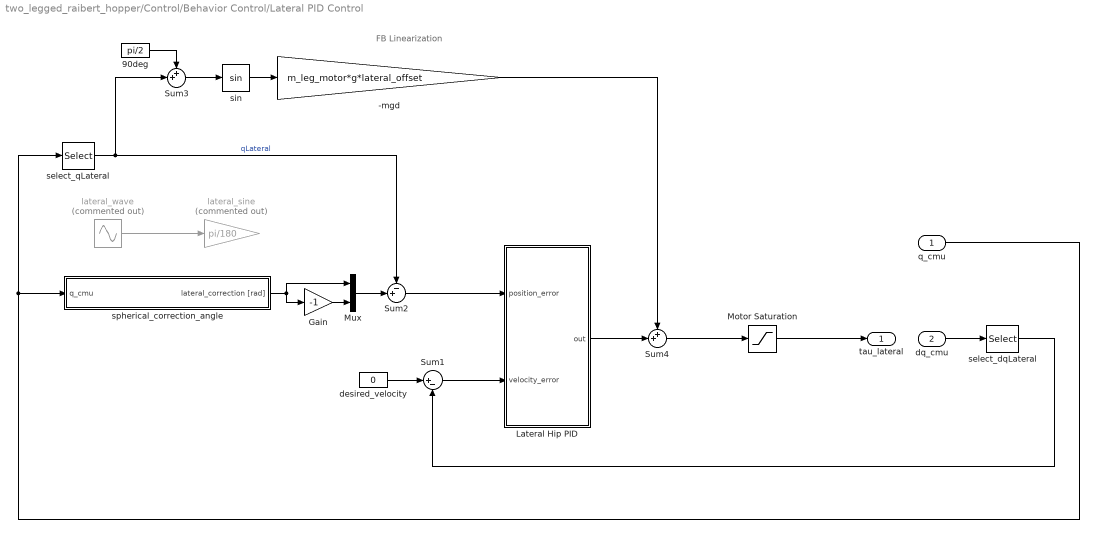
== system two_legged_raibert_hopper/Control/Behavior Control/Lateral PID Control ==
  note: FB Linearization
  q_cmu : Inport
  dq_cmu : Inport  Port=2
  -mgd : Gain  Gain=m_leg_motor*g*lateral_offset
  90deg : Constant  Value=pi/2
  Gain : Gain  Gain=-1
  Lateral Hip PID : Subsystem
  Motor Saturation : Saturate  UpperLimit=max_torque_lateral  LowerLimit=-max_torque_lateral
      settings: AttributesFormatString=Top: %<UpperLimit>\nBottom: %<LowerLimit>
  Mux : Mux  Inputs=2
  Sum1 : Sum  Inputs=|+-
  Sum2 : Sum  Inputs=-+|
  Sum3 : Sum  Inputs=++|
  Sum4 : Sum  Inputs=++|
  desired_velocity : Constant  Value=0
  lateral_sine : Gain  Commented=on  Gain=pi/180
  lateral_wave : Sin  Commented=on  Amplitude=5  Frequency=2*pi*(1/2)  SampleTime=0
  select_dqLateral : Selector  InputPortWidth=13  Indices=[9 10]
  select_qLateral : Selector  InputPortWidth=13  Indices=[9 10]
  sin : Trigonometry
  spherical_correction_angle : Subsystem
  tau_lateral : Outport
  wires:
  lateral_wave/1 -> lateral_sine/1
  Lateral Hip PID/1(out) -> Sum4/2
  Sum2/1 -> Lateral Hip PID/1(position_error)
  q_cmu/1 -> spherical_correction_angle/1(q_cmu), select_qLateral/1
  select_dqLateral/1 -> Sum1/2
  dq_cmu/1 -> select_dqLateral/1
  Sum4/1 -> Motor Saturation/1
  desired_velocity/1 -> Sum1/1
  Sum1/1 -> Lateral Hip PID/2(velocity_error)
  Gain/1 -> Mux/2
  Mux/1 -> Sum2/2
  select_qLateral/1 -> Sum3/2, Sum2/1  "qLateral"
  Motor Saturation/1 -> tau_lateral/1
  spherical_correction_angle/1(lateral_correction [rad]) -> Mux/1, Gain/1
  -mgd/1 -> Sum4/1
  Sum3/1 -> sin/1
  90deg/1 -> Sum3/1
  sin/1 -> -mgd/1

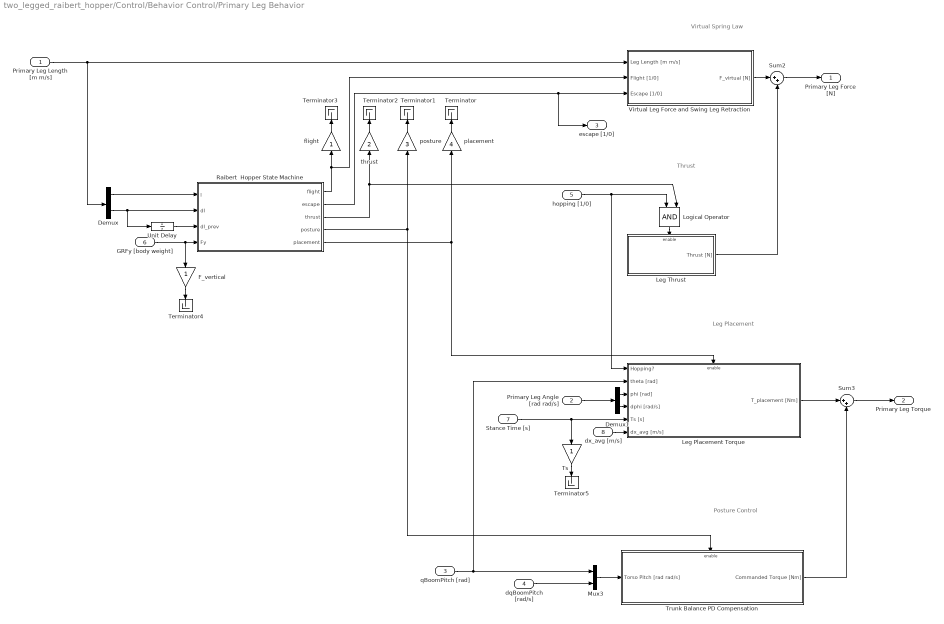
== system two_legged_raibert_hopper/Control/Behavior Control/Primary Leg Behavior ==
  note: Virtual Spring Law
  note: Thrust
  note: Posture Control
  note: Leg Placement
  Primary Leg Length [m m/s] : Inport
  Primary Leg Angle [rad rad/s] : Inport  Port=2
  qBoomPitch [rad] : Inport  Port=3
  dqBoomPitch [rad/s] : Inport  Port=4
  hopping [1/0] : Inport  Port=5
  GRFy [body weight] : Inport  Port=6
  Stance Time [s] : Inport  Port=7
  dx_avg [m/s] : Inport  Port=8
  Demux : Demux  Outputs=2
  Demux1 : Demux  Outputs=2
  F_vertical : Gain
  Leg Placement Torque : Subsystem
  Leg Thrust : Subsystem
  Logical Operator : Logic  IconShape=distinctive  AllPortsSameDT=off  OutDataTypeStr=boolean
  Mux3 : Mux  Inputs=2
  Raibert  Hopper State Machine : State Transition Table  TreatAsAtomicUnit=on
  Sum2 : Sum  Inputs=|++
  Sum3 : Sum  Inputs=|++
  Terminator{,1..5} (6 alike) : Terminator
  Trunk Balance PD Compensation : Subsystem
  Ts : Gain
  Unit Delay : UnitDelay  SampleTime=-1
  Virtual Leg Force and Swing Leg Retraction : Subsystem
  flight : Gain
  placement : Gain  Gain=4
  posture : Gain  Gain=3
  thrust : Gain  Gain=2
  Primary Leg Force [N] : Outport
  Primary Leg Torque : Outport  Port=2
  escape [1/0] : Outport  Port=3
  wires:
  Raibert  Hopper State Machine/4(posture) -> Trunk Balance PD Compensation/Enable, posture/1
  Mux3/1 -> Trunk Balance PD Compensation/1(Torso Pitch [rad rad/s])
  qBoomPitch [rad]/1 -> Mux3/1, Leg Placement Torque/2(theta [rad])
  dqBoomPitch [rad/s]/1 -> Mux3/2
  Trunk Balance PD Compensation/1(Commanded Torque [Nm]) -> Sum3/2
  Unit Delay/1 -> Raibert  Hopper State Machine/3(dl_prev)
  GRFy [body weight]/1 -> F_vertical/1, Raibert  Hopper State Machine/4(Fy)
  Demux/2 -> Unit Delay/1, Raibert  Hopper State Machine/2(dl)
  Raibert  Hopper State Machine/3(thrust) -> Logical Operator/2, thrust/1
  Leg Thrust/1(Thrust [N]) -> Sum2/2
  Sum2/1 -> Primary Leg Force [N]/1
  Raibert  Hopper State Machine/1(flight) -> flight/1, Virtual Leg Force and Swing Leg Retraction/2(Flight [1/0])
  Virtual Leg Force and Swing Leg Retraction/1(F_virtual [N]) -> Sum2/1
  Raibert  Hopper State Machine/2(escape) -> escape [1/0]/1, Virtual Leg Force and Swing Leg Retraction/3(Escape [1/0])
  Leg Placement Torque/1(T_placement [Nm]) -> Sum3/1
  Sum3/1 -> Primary Leg Torque/1
  dx_avg [m/s]/1 -> Leg Placement Torque/6(dx_avg [m/s])
  Demux1/1 -> Leg Placement Torque/3(phi [rad])
  Demux1/2 -> Leg Placement Torque/4(dphi [rad/s])
  Primary Leg Angle [rad rad/s]/1 -> Demux1/1
  Stance Time [s]/1 -> Leg Placement Torque/5(Ts [s]), Ts/1
  Raibert  Hopper State Machine/5(placement) -> Leg Placement Torque/Enable, placement/1
  Logical Operator/1 -> Leg Thrust/Enable
  placement/1 -> Terminator/1
  posture/1 -> Terminator1/1
  thrust/1 -> Terminator2/1
  Primary Leg Length [m m/s]/1 -> Demux/1, Virtual Leg Force and Swing Leg Retraction/1(Leg Length [m m/s])
  F_vertical/1 -> Terminator4/1
  flight/1 -> Terminator3/1
  Demux/1 -> Raibert  Hopper State Machine/1(l)
  Ts/1 -> Terminator5/1
  hopping [1/0]/1 -> Leg Placement Torque/1(Hopping?), Logical Operator/1

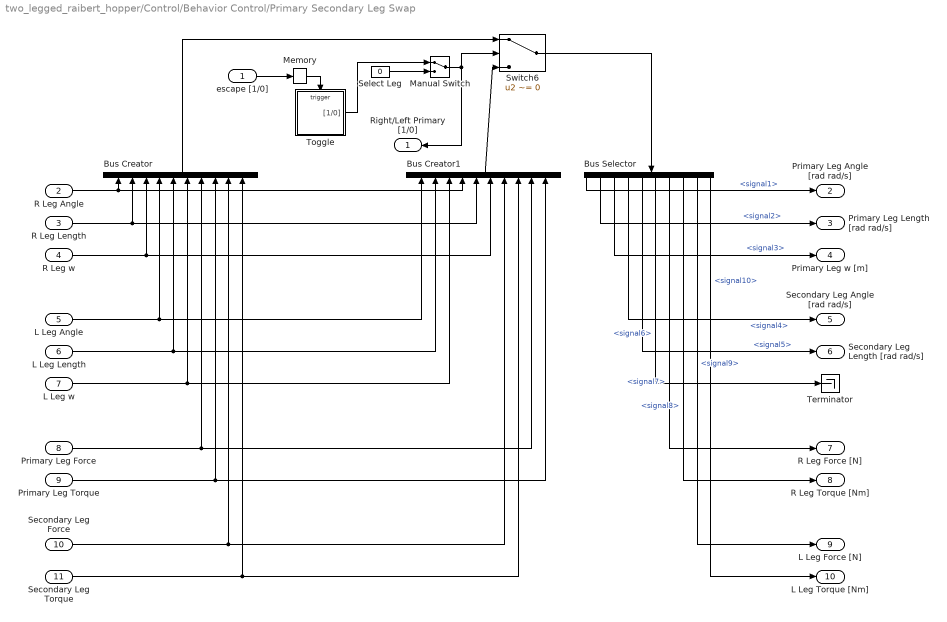
== system two_legged_raibert_hopper/Control/Behavior Control/Primary Secondary Leg Swap ==
  escape [1/0] : Inport
  R Leg Angle : Inport  Port=2
  R Leg Length : Inport  Port=3
  R Leg w : Inport  Port=4
  L Leg Angle : Inport  Port=5
  L Leg Length : Inport  Port=6
  L Leg w : Inport  Port=7
  Primary Leg Force : Inport  Port=8
  Primary Leg Torque : Inport  Port=9
  Secondary Leg Force : Inport  Port=10
  Secondary Leg Torque : Inport  Port=11
  Bus Creator : BusCreator  Inputs=10
  Bus Creator1 : BusCreator  Inputs=10
  Bus Selector : BusSelector  OutputSignals=signal1,signal2,signal3,signal4,signal5,signal6,signal7,signal8,signal9,signal10
  Manual Switch : ManualSwitch
  Memory : Memory  InheritSampleTime=on
  Select Leg : Constant  Value=0  OutDataTypeStr=boolean
  Switch6 : Switch  Criteria=u2 ~= 0  ZeroCross=off
  Terminator : Terminator
  Toggle : Subsystem
  Right/Left Primary [1/0] : Outport
  Primary Leg Angle [rad rad/s] : Outport  Port=2
  Primary Leg Length [rad rad/s] : Outport  Port=3
  Primary Leg w [m] : Outport  Port=4
  Secondary Leg Angle [rad rad/s] : Outport  Port=5
  Secondary Leg Length [rad rad/s] : Outport  Port=6
  R Leg Force [N] : Outport  Port=7
  R Leg Torque [Nm] : Outport  Port=8
  L Leg Force [N] : Outport  Port=9
  L Leg Torque [Nm] : Outport  Port=10
  wires:
  Switch6/1 -> Bus Selector/1
  Bus Creator1/1 -> Switch6/3
  Bus Creator/1 -> Switch6/1
  Primary Leg Torque/1 -> Bus Creator1/10, Bus Creator/8
  Secondary Leg Torque/1 -> Bus Creator1/8, Bus Creator/10
  Secondary Leg Force/1 -> Bus Creator1/7, Bus Creator/9
  escape [1/0]/1 -> Memory/1
  R Leg Length/1 -> Bus Creator1/5, Bus Creator/2
  L Leg w/1 -> Bus Creator/6, Bus Creator1/3
  R Leg Angle/1 -> Bus Creator1/4, Bus Creator/1
  R Leg w/1 -> Bus Creator1/6, Bus Creator/3
  Primary Leg Force/1 -> Bus Creator1/9, Bus Creator/7
  L Leg Length/1 -> Bus Creator/5, Bus Creator1/2
  L Leg Angle/1 -> Bus Creator/4, Bus Creator1/1
  Bus Selector/1 -> Primary Leg Angle [rad rad/s]/1  "<signal1>"
  Bus Selector/2 -> Primary Leg Length [rad rad/s]/1  "<signal2>"
  Bus Selector/3 -> Primary Leg w [m]/1  "<signal3>"
  Bus Selector/4 -> Secondary Leg Angle [rad rad/s]/1  "<signal4>"
  Bus Selector/5 -> Secondary Leg Length [rad rad/s]/1  "<signal5>"
  Bus Selector/6 -> Terminator/1  "<signal6>"
  Bus Selector/7 -> R Leg Force [N]/1  "<signal7>"
  Bus Selector/8 -> R Leg Torque [Nm]/1  "<signal8>"
  Bus Selector/9 -> L Leg Force [N]/1  "<signal9>"
  Bus Selector/10 -> L Leg Torque [Nm]/1  "<signal10>"
  Select Leg/1 -> Manual Switch/2
  Manual Switch/1 -> Switch6/2, Right/Left Primary [1/0]/1
  Toggle/1("[1/0]") -> Manual Switch/1
  Memory/1 -> Toggle/Trigger

== system two_legged_raibert_hopper/Control/Behavior Control/R Leg Calculator ==
  Front [rad rad/s] : Inport
  Back [rad rad/s] : Inport  Port=2
  Demux1 : Demux  Outputs=2
  Gain1 : Gain  Gain=2*l_seg
  Gain2 : Gain  Gain=l_seg
  Gain3 : Gain  Gain=-1
  Gain4 : Gain  Gain=0.5
  Gain5 : Gain  Gain=0.5
  Gain6 : Gain  Gain=2
  Mux1 : Mux  Inputs=2
  Product : Product  RndMeth=Zero
  Sum4 : Sum  Inputs=+|+
  Sum5 : Sum  Inputs=+|-
  Trigonometric Function : Trigonometry  Operator=cos
  Trigonometric Function1 : Trigonometry
  "Leg Length [m m/s] " : Outport
  Leg Angle [rad rad/s] : Outport  Port=2
  Leg Splay [rad rad/s] : Outport  Port=3
  w [m] : Outport  Port=4
  wires:
  Gain6/1 -> w [m]/1
  Gain4/1 -> Trigonometric Function1/1, Trigonometric Function/1
  Trigonometric Function/1 -> Gain1/1
  Gain1/1 -> Mux1/1
  Trigonometric Function1/1 -> Gain2/1
  Product/1 -> Mux1/2
  Front [rad rad/s]/1 -> Sum5/2, Sum4/2
  Back [rad rad/s]/1 -> Sum4/1, Sum5/1
  Demux1/2 -> Gain3/1
  Gain3/1 -> Product/2
  Demux1/1 -> Gain4/1
  Gain2/1 -> Product/1, Gain6/1
  Sum5/1 -> Leg Splay [rad rad/s]/1, Demux1/1
  Mux1/1 -> "Leg Length [m m/s] "/1
  Sum4/1 -> Gain5/1
  Gain5/1 -> Leg Angle [rad rad/s]/1

== system two_legged_raibert_hopper/Control/Behavior Control/Raibert Initiated ==
  Enable : EnablePort  StatesWhenEnabling=reset
  Constant : Constant
  Hopping? : Outport  InitialOutput=[0]
  wires:
  Constant/1 -> Hopping?/1

== system two_legged_raibert_hopper/Control/Behavior Control/Secondary Leg Behavior ==
  Secondary Leg Angle [rad rad/s] : Inport
  Secondary Leg Length [m m/s] : Inport  Port=2
  Primary Leg Angle [rad rad/s] : Inport  Port=3
  Torso Pitch [rad rad/s] : Inport  Port=4
  Constant12 : Constant  Value=0.75
  Constant9 : Constant  Value=0
  Demux5 : Demux  Outputs=2
  Fcn2 : Fcn  Expr=2*pi-u(1)
  Leg Angle PD : Subsystem
  Leg Length PD : Subsystem
  Sum2 : Sum  Inputs=|++
  k_virtual6 : Gain  Gain=-1
  Secondary Leg Force [N] : Outport
  Secondary Leg Torque [Nm] : Outport  Port=2
  wires:
  Constant9/1 -> Leg Length PD/2(Desired Velocity)
  Constant12/1 -> Leg Length PD/1(Desired Length)
  Secondary Leg Length [m m/s]/1 -> Leg Length PD/3(Leg Length [m m/s])
  Leg Length PD/1(Commanded Force [N]) -> Secondary Leg Force [N]/1
  Secondary Leg Angle [rad rad/s]/1 -> Sum2/1
  Torso Pitch [rad rad/s]/1 -> Sum2/2
  Sum2/1 -> Leg Angle PD/3(Leg Angle [rad rad/s])
  Fcn2/1 -> Leg Angle PD/1(Desired Angle)
  k_virtual6/1 -> Leg Angle PD/2(Desired Velocity)
  Primary Leg Angle [rad rad/s]/1 -> Demux5/1
  Demux5/1 -> Fcn2/1
  Demux5/2 -> k_virtual6/1
  Leg Angle PD/1(Commanded Leg Torque [Nm]) -> Secondary Leg Torque [Nm]/1

== system two_legged_raibert_hopper/Control/Behavior Control/Torque Distribution Left ==
  Leg Torque [Nm] : Inport
  Leg Force [N] : Inport  Port=2
  w [m] : Inport  Port=3
  Gain : Gain  Gain=0.5
  Gain1 : Gain  Gain=0.5
  Motor Torque Saturation Optimization : MATLAB Function  TreatAsAtomicUnit=on
  Product : Product  RndMeth=Zero
  Sum : Sum  Inputs=|++
  Sum1 : Sum  Inputs=+-|
  Back Torque [Nm] : Outport
  Front Torque [Nm] : Outport  Port=2
  wires:
  Gain/1 -> Motor Torque Saturation Optimization/1(x1s)
  Gain1/1 -> Motor Torque Saturation Optimization/2(x2s)
  Product/1 -> Gain1/1
  Leg Force [N]/1 -> Product/1
  Motor Torque Saturation Optimization/2(t2) -> Sum/2, Sum1/2
  w [m]/1 -> Product/2
  Motor Torque Saturation Optimization/1(t1) -> Sum1/1, Sum/1
  Sum/1 -> Front Torque [Nm]/1
  Leg Torque [Nm]/1 -> Gain/1
  Sum1/1 -> Back Torque [Nm]/1

== system two_legged_raibert_hopper/Control/Behavior Control/Torque Distribution Right ==
  Leg Torque [Nm] : Inport
  Leg Force [N] : Inport  Port=2
  w [m] : Inport  Port=3
  Gain : Gain  Gain=0.5
  Gain1 : Gain  Gain=0.5
  Motor Torque Saturation Optimization : MATLAB Function  TreatAsAtomicUnit=on
  Product : Product  RndMeth=Zero
  Sum : Sum  Inputs=|++
  Sum1 : Sum  Inputs=+-|
  Back Torque [Nm] : Outport
  Front Torque [Nm] : Outport  Port=2
  wires:
  Sum1/1 -> Back Torque [Nm]/1
  Leg Torque [Nm]/1 -> Gain/1
  Sum/1 -> Front Torque [Nm]/1
  Motor Torque Saturation Optimization/1(t1) -> Sum/1, Sum1/1
  w [m]/1 -> Product/2
  Motor Torque Saturation Optimization/2(t2) -> Sum1/2, Sum/2
  Leg Force [N]/1 -> Product/1
  Product/1 -> Gain1/1
  Gain1/1 -> Motor Torque Saturation Optimization/2(x2s)
  Gain/1 -> Motor Torque Saturation Optimization/1(x1s)

== system two_legged_raibert_hopper/Control/Behavior Control/Velocity Estimation ==
  qRoll [rad] : Inport
  dqYaw [rad/s] : Inport  Port=2
  dqPitch [rad/s] : Inport  Port=3
  Recursive Moving Average : Subsystem
  dx_from_yaw_and_roll : MATLAB Function  TreatAsAtomicUnit=on
  dx_avg [m/s] : Outport
  wires:
  Recursive Moving Average/1(dx_avg [m/s]) -> dx_avg [m/s]/1
  dx_from_yaw_and_roll/1(dx) -> Recursive Moving Average/1(dx [m/s])
  dqYaw [rad/s]/1 -> dx_from_yaw_and_roll/2(dqYaw)
  qRoll [rad]/1 -> dx_from_yaw_and_roll/1(qRoll)
  dqPitch [rad/s]/1 -> dx_from_yaw_and_roll/3(dqPitch)

== system two_legged_raibert_hopper/Control/Actuator Control/SEA Controller (Torque)/Antiresonance Compensation ==
  Torque : Inport
  Notch Filter (Flight) : DiscreteTransferFcn  Numerator=[K_notch_f1 K_notch_f1*A1_notch_f1 K_notch_f1*A2_notch_f1]  Denominator=[1 B1_notch_f1 B2_notch_f1]  SampleTime=sample_time
  Filtered Torque : Outport
  wires:
  Torque/1 -> Notch Filter (Flight)/1
  Notch Filter (Flight)/1 -> Filtered Torque/1

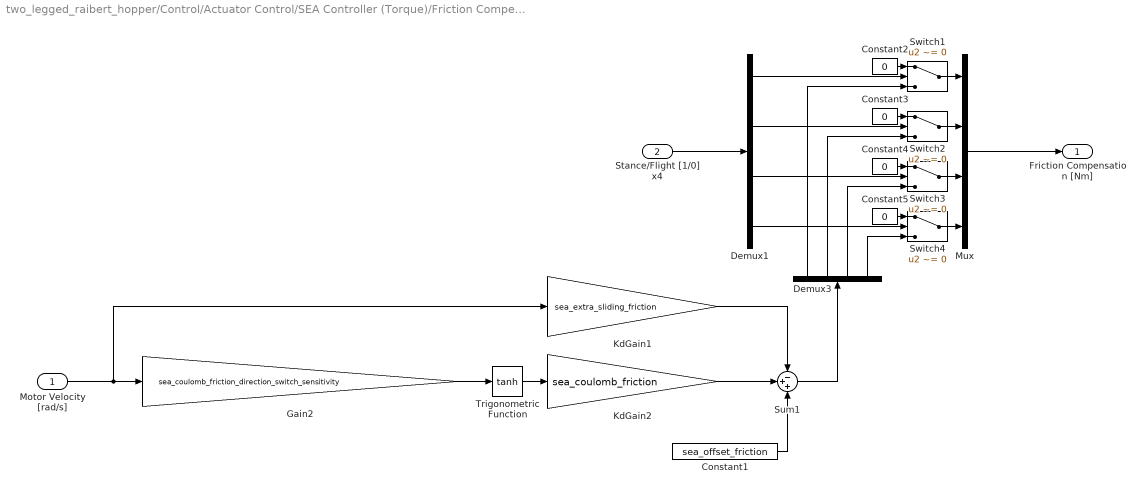
== system two_legged_raibert_hopper/Control/Actuator Control/SEA Controller (Torque)/Friction Compensation ==
  Motor Velocity [rad/s] : Inport
  Stance/Flight [1/0] x4 : Inport  Port=2
  Constant1 : Constant  Value=sea_offset_friction
  Constant{2..5} (4 alike) : Constant  Value=0
  Demux1 : Demux
  Demux3 : Demux
  Gain2 : Gain  Gain=sea_coulomb_friction_direction_switch_sensitivity
  KdGain1 : Gain  Description=xPCTag(1)=kd_sea_torque;  Gain=sea_extra_sliding_friction
  KdGain2 : Gain  Description=xPCTag(1)=kd_sea_torque;  Gain=sea_coulomb_friction
  Mux : Mux
  Sum1 : Sum  Inputs=-++
  Switch{1..4} (4 alike) : Switch  Criteria=u2 ~= 0
  Trigonometric Function : Trigonometry  Operator=tanh
  Friction Compensation [Nm] : Outport
  wires:
  Sum1/1 -> Demux3/1
  Constant5/1 -> Switch4/1
  Constant4/1 -> Switch3/1
  Constant3/1 -> Switch2/1
  Constant2/1 -> Switch1/1
  Stance/Flight [1/0] x4/1 -> Demux1/1
  Demux3/1 -> Switch1/3
  Demux3/2 -> Switch2/3
  Demux3/3 -> Switch3/3
  Demux3/4 -> Switch4/3
  Demux1/1 -> Switch1/2
  Switch1/1 -> Mux/1
  Switch4/1 -> Mux/4
  Switch3/1 -> Mux/3
  Switch2/1 -> Mux/2
  Demux1/2 -> Switch2/2
  Demux1/3 -> Switch3/2
  Demux1/4 -> Switch4/2
  Constant1/1 -> Sum1/3
  KdGain2/1 -> Sum1/2
  Motor Velocity [rad/s]/1 -> KdGain1/1, Gain2/1
  Gain2/1 -> Trigonometric Function/1
  Trigonometric Function/1 -> KdGain2/1
  Mux/1 -> Friction Compensation [Nm]/1
  KdGain1/1 -> Sum1/1

== system two_legged_raibert_hopper/Control/Actuator Control/SEA Controller (Torque)/Loaded Unloaded Switch ==
  Loaded Signal : Inport
  Loaded/Unloaded [1/0] x4 : Inport  Port=2
  Unloaded Signal : Inport  Port=3
  Demux : Demux
  Demux1 : Demux
  Demux2 : Demux
  Mux : Mux
  Switch{,1..3} (4 alike) : Switch  Criteria=u2 ~= 0
  Signal : Outport
  wires:
  Demux/4 -> Switch3/2
  Demux/3 -> Switch2/2
  Demux/2 -> Switch1/2
  Switch1/1 -> Mux/2
  Switch2/1 -> Mux/3
  Switch3/1 -> Mux/4
  Loaded/Unloaded [1/0] x4/1 -> Demux/1
  Mux/1 -> Signal/1
  Switch/1 -> Mux/1
  Demux/1 -> Switch/2
  Loaded Signal/1 -> Demux1/1
  Demux1/1 -> Switch/1
  Demux1/2 -> Switch1/1
  Demux1/3 -> Switch2/1
  Demux1/4 -> Switch3/1
  Unloaded Signal/1 -> Demux2/1
  Demux2/4 -> Switch3/3
  Demux2/3 -> Switch2/3
  Demux2/2 -> Switch1/3
  Demux2/1 -> Switch/3

== system two_legged_raibert_hopper/Control/Actuator Control/SEA Controller (Torque)/Stance Flight Kd Switch ==
  Kd Stance : Inport
  Stance/Flight [1/0] x4 : Inport  Port=2
  Kd Flight : Inport  Port=3
  Demux : Demux
  Demux1 : Demux
  Demux2 : Demux
  Mux : Mux
  Switch{,1..3} (4 alike) : Switch  Criteria=u2 ~= 0
  Kd : Outport
  wires:
  Demux2/1 -> Switch/3
  Demux2/2 -> Switch1/3
  Demux2/3 -> Switch2/3
  Demux2/4 -> Switch3/3
  Kd Flight/1 -> Demux2/1
  Demux1/4 -> Switch3/1
  Demux1/3 -> Switch2/1
  Demux1/2 -> Switch1/1
  Demux1/1 -> Switch/1
  Kd Stance/1 -> Demux1/1
  Demux/1 -> Switch/2
  Switch/1 -> Mux/1
  Mux/1 -> Kd/1
  Stance/Flight [1/0] x4/1 -> Demux/1
  Switch3/1 -> Mux/4
  Switch2/1 -> Mux/3
  Switch1/1 -> Mux/2
  Demux/2 -> Switch1/2
  Demux/3 -> Switch2/2
  Demux/4 -> Switch3/2

== system two_legged_raibert_hopper/Control/Actuator Control/SEA Controller (Torque)/Stance Flight Kp Switch ==
  Kp Stance : Inport
  Stance/Flight [1/0] x4 : Inport  Port=2
  Kp Flight : Inport  Port=3
  Demux : Demux
  Mux : Mux
  Switch{,1..3} (4 alike) : Switch  Criteria=u2 ~= 0
  Kp : Outport
  wires:
  Demux/4 -> Switch3/2
  Demux/3 -> Switch2/2
  Demux/2 -> Switch1/2
  Switch1/1 -> Mux/2
  Switch2/1 -> Mux/3
  Switch3/1 -> Mux/4
  Stance/Flight [1/0] x4/1 -> Demux/1
  Mux/1 -> Kp/1
  Switch/1 -> Mux/1
  Demux/1 -> Switch/2
  Kp Stance/1 -> Switch/1, Switch1/1, Switch2/1, Switch3/1
  Kp Flight/1 -> Switch1/3, Switch2/3, Switch3/3, Switch/3

== system two_legged_raibert_hopper/Control/Actuator Control/SEA Controller (Torque)/dtau_des ==
  x : Inport
  Gain1 : Gain  Gain=1/sample_time
  difference : simulink/Discrete/Difference  ICPrevInput=0.0  InputProcessing=Inherited  OutMin=[]  OutMax=[]  OutDataType=fixdt(1, 16)  OutScaling=2^-10  DoSatur=off
  two_pole_filter : DiscreteTransferFcn  Numerator=[A_lpf_dtau 0 0]  Denominator=[1 B1_lpf_dtau B2_lpf_dtau]  SampleTime=sample_time
  dx/dt : Outport
  wires:
  Gain1/1 -> difference/1
  difference/1 -> two_pole_filter/1
  x/1 -> Gain1/1
  two_pole_filter/1 -> dx/dt/1

== system two_legged_raibert_hopper/Control/Actuator Control/SEA Controller (Torque)/filtered_derivative ==
  x : Inport
  Gain1 : Gain  Gain=1/sample_time
  difference : simulink/Discrete/Difference  ICPrevInput=0.0  InputProcessing=Inherited  OutMin=[]  OutMax=[]  OutDataType=fixdt(1, 16)  OutScaling=2^-10  DoSatur=off
  two_pole_filter : DiscreteTransferFcn  Numerator=[A_lpf_accel 0 0]  Denominator=[1 B1_lpf_accel B2_lpf_accel]  SampleTime=sample_time
  dx/dt : Outport
  wires:
  two_pole_filter/1 -> dx/dt/1
  x/1 -> Gain1/1
  difference/1 -> two_pole_filter/1
  Gain1/1 -> difference/1

== system two_legged_raibert_hopper/Control/Behavior Control/Contact Estimation/Contact Time ==
  Enable : EnablePort  StatesWhenEnabling=reset  ShowOutputPort=on
  Constant : Constant
  Discrete-Time Integrator : DiscreteIntegrator  IntegratorMethod=Accumulation: Forward Euler  gainval=sample_time  ExternalReset=rising  SampleTime=sample_time  ICPrevOutput=DiscIntNeverNeededParam  ICPrevScaledInput=DiscIntNeverNeededParam
  ts [s] : Outport  InitialOutput=[0]
  wires:
  Constant/1 -> Discrete-Time Integrator/1
  Enable/1 -> Discrete-Time Integrator/2
  Discrete-Time Integrator/1 -> ts [s]/1

== system two_legged_raibert_hopper/Control/Behavior Control/Contact Estimation/Last Contact Time ==
  ts [s] : Inport
  Trigger : TriggerPort  TriggerType=falling  PortDimensions=1
  Ts [s] : Outport  InitialOutput=[initial_dt]
  wires:
  ts [s]/1 -> Ts [s]/1

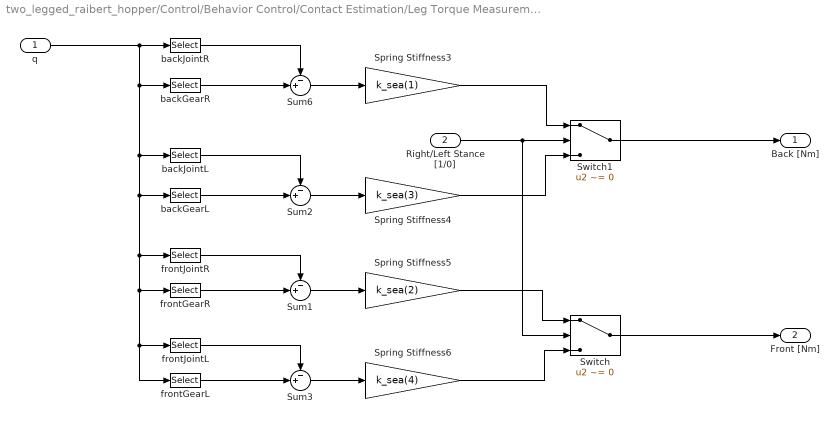
== system two_legged_raibert_hopper/Control/Behavior Control/Contact Estimation/Leg Torque Measurements ==
  q : Inport
  Right/Left Stance [1/0] : Inport  Port=2
  Spring Stiffness3 : Gain  Gain=k_sea(1)
  Spring Stiffness4 : Gain  Gain=k_sea(3)
  Spring Stiffness5 : Gain  Gain=k_sea(2)
  Spring Stiffness6 : Gain  Gain=k_sea(4)
  Sum{1..3,6} (4 alike) : Sum  Inputs=-+|
  Switch : Switch  Criteria=u2 ~= 0
  Switch1 : Switch  Criteria=u2 ~= 0
  backGearL : Selector  InputPortWidth=13  Indices=[6]
  backGearR : Selector  InputPortWidth=13  Indices=[2]
  backJointL : Selector  InputPortWidth=13  Indices=[5]
  backJointR : Selector  InputPortWidth=13  Indices=[1]
  frontGearL : Selector  InputPortWidth=13  Indices=[8]
  frontGearR : Selector  InputPortWidth=13  Indices=[4]
  frontJointL : Selector  InputPortWidth=13  Indices=[7]
  frontJointR : Selector  InputPortWidth=13  Indices=[3]
  Back [Nm] : Outport
  Front [Nm] : Outport  Port=2
  wires:
  Right/Left Stance [1/0]/1 -> Switch1/2, Switch/2
  Sum3/1 -> Spring Stiffness6/1
  Sum2/1 -> Spring Stiffness4/1
  Switch1/1 -> Back [Nm]/1
  backJointL/1 -> Sum2/1
  frontGearL/1 -> Sum3/2
  frontJointL/1 -> Sum3/1
  backGearL/1 -> Sum2/2
  Sum6/1 -> Spring Stiffness3/1
  Sum1/1 -> Spring Stiffness5/1
  Switch/1 -> Front [Nm]/1
  backJointR/1 -> Sum6/1
  frontGearR/1 -> Sum1/2
  frontJointR/1 -> Sum1/1
  backGearR/1 -> Sum6/2
  q/1 -> backGearR/1, backJointL/1, backGearL/1, frontJointR/1, frontGearR/1, frontJointL/1, frontGearL/1, backJointR/1
  Spring Stiffness3/1 -> Switch1/1
  Spring Stiffness4/1 -> Switch1/3
  Spring Stiffness5/1 -> Switch/1
  Spring Stiffness6/1 -> Switch/3

== system two_legged_raibert_hopper/Control/Behavior Control/Contact Estimation/Vertical Spring Force ==
  theta [rad] : Inport
  phi [rad] : Inport  Port=2
  Force [N] : Inport  Port=3
  Gain : Gain  Gain=-1
  Product : Product
  Sum : Sum  Inputs=++|
  Trigonometric Function : Trigonometry  Operator=cos
  Vertical Force [N] : Outport
  wires:
  Force [N]/1 -> Product/1
  phi [rad]/1 -> Sum/2
  theta [rad]/1 -> Sum/1
  Trigonometric Function/1 -> Product/2
  Product/1 -> Gain/1
  Sum/1 -> Trigonometric Function/1
  Gain/1 -> Vertical Force [N]/1

== system two_legged_raibert_hopper/Control/Behavior Control/Lateral PID Control/Lateral Hip PID ==
  position_error : Inport
  velocity_error : Inport  Port=2
  Discrete-Time Integrator : DiscreteIntegrator  IntegratorMethod=Integration: Trapezoidal  SampleTime=sample_time  LimitOutput=on  UpperSaturationLimit=i_limit_lateral  LowerSaturationLimit=-i_limit_lateral  ICPrevOutput=DiscIntNeverNeededParam  ICPrevScaledInput=DiscIntNeverNeededParam
  Sum : Sum  Inputs=+++
  kd_lateral : Gain  Description=xPCTag(1)=kd_lateral;  Gain=kd_lateral
  ki_lateral : Gain  Description=xPCTag(1)=ki_lateral;  Gain=ki_lateral
  kp_lateral : Gain  Description=xPCTag(1)=kp_lateral;  Gain=kp_lateral
  out : Outport
  wires:
  velocity_error/1 -> kd_lateral/1
  Discrete-Time Integrator/1 -> Sum/3
  ki_lateral/1 -> Discrete-Time Integrator/1
  kp_lateral/1 -> Sum/2
  position_error/1 -> ki_lateral/1, kp_lateral/1
  Sum/1 -> out/1
  kd_lateral/1 -> Sum/1
